simulink model "opgave2Johan"  (R2023b)
settings: Solver=VariableStepAuto  StartTime=0.0  StopTime=10.0  RelTol=1e-3
libraries: dspsrcs4 x2
settings Model: Creator=theil  LastModifiedBy=theil

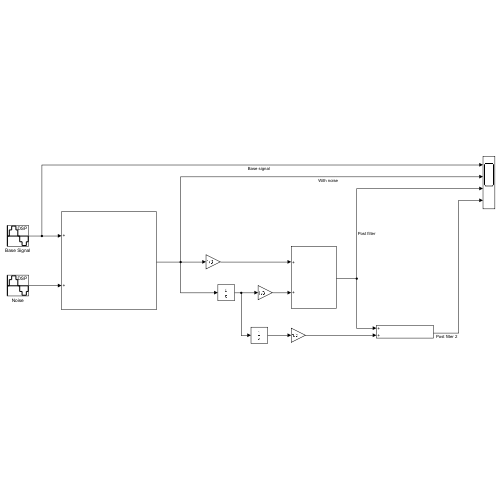
[thumbnail: Simulink's stored preview of the top-level diagram]
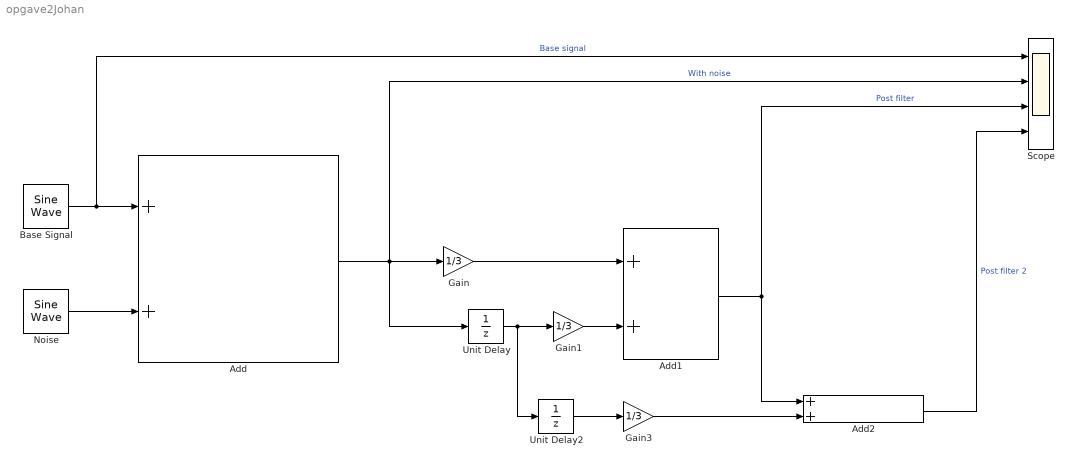
== system opgave2Johan ==
  Add : Sum
  Add1 : Sum
  Add2 : Sum
  Base Signal : dspsrcs4/Sine Wave  Amplitude=10  Frequency=1/(2*pi)  Phase=0  SampleMode=Discrete  OutComplex=Real  CompMethod=Trigonometric fcn  TableSize=Speed  SampleTime=0.2  SamplesPerFrame=1  ResetState=Restart at time zero  OutputFrames=off  dataType=double  wordLen=16  udDataType=sfix(16)  fracBitsMode=Best precision  numFracBits=15  OutDataTypeStr=double  LastOutDataTypeStr=double
  Gain : Gain  Gain=1/3
  Gain1 : Gain  Gain=1/3
  Gain3 : Gain  Gain=1/3
  Noise : dspsrcs4/Sine Wave  Amplitude=2.5  Frequency=18/(2*pi)  Phase=0  SampleMode=Discrete  OutComplex=Real  CompMethod=Trigonometric fcn  TableSize=Speed  SampleTime=0.2  SamplesPerFrame=1  ResetState=Restart at time zero  OutputFrames=off  dataType=double  wordLen=16  udDataType=sfix(16)  fracBitsMode=Best precision  numFracBits=15  OutDataTypeStr=double  LastOutDataTypeStr=double
  Scope : Scope  NumInputPorts=4
  Unit Delay : UnitDelay  SampleTime=-1  HasFrameUpgradeWarning=on
  Unit Delay2 : UnitDelay  SampleTime=-1  HasFrameUpgradeWarning=on
  wires:
  Noise/1 -> Add/2
  Base Signal/1 -> Add/1, Scope/1  "Base signal"
  Add/1 -> Scope/2, Unit Delay/1, Gain/1  "With noise"
  Unit Delay/1 -> Unit Delay2/1, Gain1/1
  Gain1/1 -> Add1/2
  Gain/1 -> Add1/1
  Add1/1 -> Add2/1, Scope/3  "Post filter"
  Unit Delay2/1 -> Gain3/1
  Gain3/1 -> Add2/2
  Add2/1 -> Scope/4  "Post filter 2"
